simulink model "poles3_rocky"  (R2022a)
settings: Solver=VariableStepAuto  StartTime=0.0  StopTime=10.0  RelTol=1e-3
values from neighbouring files (symbols this model uses):
  a = 10.12    [poles3_calculate.m]    (also in poles5_calculate.m = 10.33; poles_calculate.m = 10.33)
  b = 0.00301    [poles3_calculate.m]    (also in poles5_calculate.m = 0.0029; poles_calculate.m = 0.0029)
  g = 9.81    [poles3_calculate.m]    (also in poles5_calculate.m; poles_calculate.m)
  Ki = real(double(solutions.Ki))    [poles3_calculate.m]    (also in poles5_calculate.m = double(solutions.Ki); poles_calculate.m = double(solutions.Ki))
  Kp = real(double(solutions.Kp))    [poles3_calculate.m]    (also in poles5_calculate.m = double(solutions.Kp); poles_calculate.m = double(solutions.Kp))
  l = 0.40038    [poles3_calculate.m]    (also in poles5_calculate.m = 0.4168; poles_calculate.m = 0.4168)
libraries: slpidlib x1
settings Model: Creator=cpark1  LastModifiedBy=cpark1

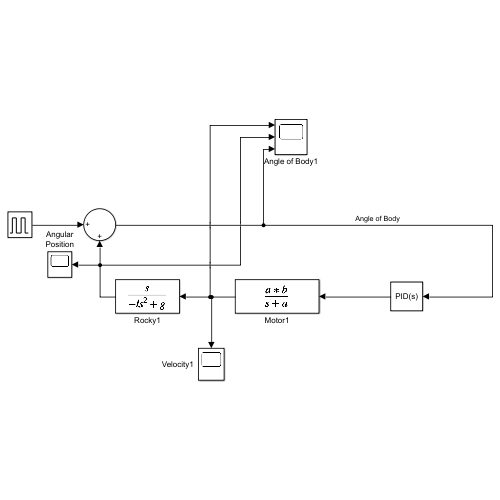
[thumbnail: Simulink's stored preview of the top-level diagram]
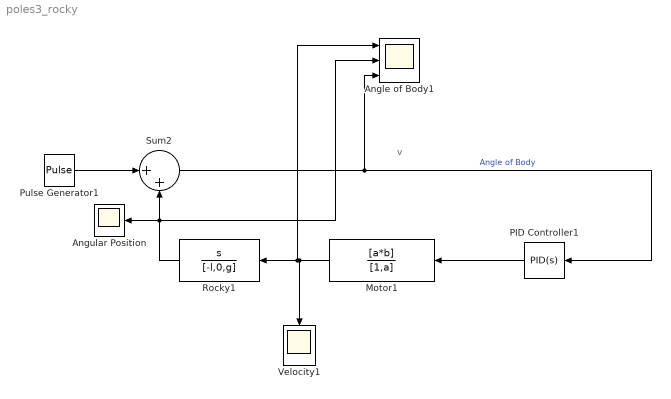
== system poles3_rocky ==
  note: v
  Angle of Body1 : Scope  NumInputPorts=3
  Angular Position : Scope
  Motor1 : TransferFcn  Numerator=[a*b]  Denominator=[1,a]  ContinuousStateAttributes='motor'
  PID Controller1 : slpidlib/PID Controller  Controller=PID  Form=Parallel  TimeDomain=Continuous-time  UseExternalTs=off  SampleTime=-1  IntegratorMethod=Forward Euler  FilterMethod=Forward Euler  ControllerParametersSource=internal  P=Kp  I=Ki  UseKiTs=off  D=0  N=100  UseFilter=on  TunerSelectOption=Transfer Function Based (PID Tuner App)  InitialConditionSource=internal  InitialConditionForIntegrator=0  InitialConditionForFilter=0  DifferentiatorICPrevScaledInput=0  ExternalReset=none  TrackingMode=off  Kt=1  LimitOutput=off  SatLimitsSource=internal  UpperSaturationLimit=inf  LowerSaturationLimit=-inf  LinearizeAsGain=on  AntiWindupMode=none  Kb=1  POutMin=[]  POutMax=[]  IOutMin=[]  IOutMax=[]  DOutMin=[]  DOutMax=[]  NOutMin=[]  NOutMax=[]  SumOutMin=[]  SumOutMax=[]  SaturationOutMin=[]  SaturationOutMax=[]  PParamMin=[]  PParamMax=[]  IParamMin=[]  IParamMax=[]  DParamMin=[]  DParamMax=[]  NParamMin=[]  NParamMax=[]  KbParamMin=[]  KbParamMax=[]  KtParamMin=[]  KtParamMax=[]  KbOutMin=[]  KbOutMax=[]  KtOutMin=[]  KtOutMax=[]  IntegratorOutMin=[]  IntegratorOutMax=[]  FilterOutMin=[]  FilterOutMax=[]  SumI1OutMin=[]  SumI1OutMax=[]  SumI2OutMin=[]  SumI2OutMax=[]  SumI3OutMin=[]  SumI3OutMax=[]  SumI4OutMin=[]  SumI4OutMax=[]  SumDOutMin=[]  SumDOutMax=[]  DifferentiatorOutMin=[]  DifferentiatorOutMax=[]  FilterDiffOutCoefMin=[]  FilterDiffOutCoefMax=[]  ReciprocalOutMin=[]  ReciprocalOutMax=[]  SumDenOutMin=[]  SumDenOutMax=[]  SumNumOutMin=[]  SumNumOutMax=[]  DivideOutMin=[]  DivideOutMax=[]  UdiffTsProdOutMin=[]  UdiffTsProdOutMax=[]  NTsProdOutMin=[]  NTsProdOutMax=[]  UintegralTsProdOutMin=[]  UintegralTsProdOutMax=[]  UngainTsProdOutMin=[]  UngainTsProdOutMax=[]  IntegratorContinuousStateAttributes=''  IntegratorStateMustResolveToSignalObject=off  IntegratorRTWStateStorageClass=Auto  FilterContinuousStateAttributes=''  FilterStateMustResolveToSignalObject=off  FilterRTWStateStorageClass=Auto  ParallelPVariant=InternalParameters  IdealPVariant=Disabled  IVariant=InternalParameters  DVariant=InternalParameters  IntegratorVariant=Continuous  SatVariant=Disabled  AWVariant=Passthrough  PCopyVariant=Disabled  TRVariant=Disabled  FdbkBlocksVariant=Forward  IdealPFdbkVariant=Disabled  SatFdbkVariant=Disabled  DerivativeFilterVariant=ContFilter  NVariant=InternalParameters  NCopyVariant=Disabled  FilterICVariant=InternalICsFilter  IntegratorICVariant=InternalICs  ExternalResetVariant=Disabled  TRSumVariant=Passthrough  SumFdbkVariant=Disabled  SumVariant=Sum_PID  TsampFilterVariant=InternalTs  TsampNgainVariant=Passthrough  TsampIntegralVariant=Passthrough  ExternalSaturationOutDataTypeStr=Inherit: Same as second input  aMode=0
  Pulse Generator1 : DiscretePulseGenerator  PulseType=Time based  Period=10  PulseWidth=5
  Rocky1 : TransferFcn  Numerator=[1,0]  Denominator=[-l,0,g]  ContinuousStateAttributes='rocky'
  Sum2 : Sum  Inputs=|++
  Velocity1 : Scope
  wires:
  Motor1/1 -> Rocky1/1, Angle of Body1/1, Velocity1/1
  Rocky1/1 -> Angle of Body1/2, Angular Position/1, Sum2/2
  Sum2/1 -> PID Controller1/1, Angle of Body1/3  "Angle of Body"
  Pulse Generator1/1 -> Sum2/1
  PID Controller1/1 -> Motor1/1
